simulink model "Stability2"  (R2024b)
settings: Solver=VariableStepAuto  StartTime=0.0  StopTime=3  RelTol=1e-3
settings Model: Creator=ADMIN  LastModifiedBy=ADMIN

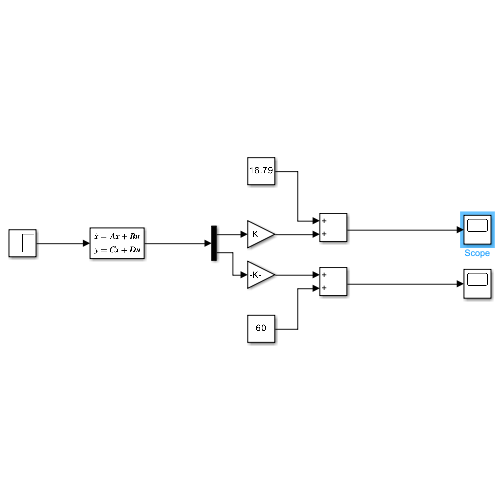
[thumbnail: Simulink's stored preview of the top-level diagram]
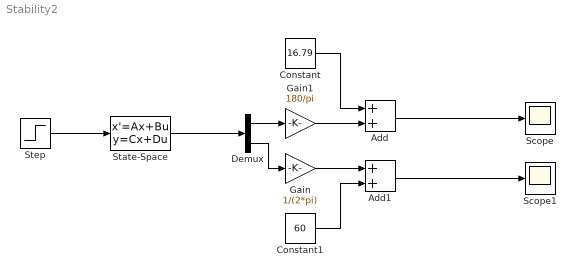
== system Stability2 ==
  Add : Sum
  Add1 : Sum
  Constant : Constant  Value=16.79
  Constant1 : Constant  Value=60
  Demux : Demux  Outputs=2
  Gain : Gain  Gain=1/(2*pi)
  Gain1 : Gain  Gain=180/pi
  Scope : Scope
  Scope1 : Scope
  State-Space : StateSpace  A=[0 1 ; -37.705 -2.617]  B=[0; 1]  C=[1 0; 0 1]  D=[0;0]  InitialCondition=0
  Step : Step  Time=0  Before=3.79  After=3.79  SampleTime=0
  wires:
  Step/1 -> State-Space/1
  Demux/1 -> Gain1/1
  State-Space/1 -> Demux/1
  Demux/2 -> Gain/1
  Gain/1 -> Add1/1
  Gain1/1 -> Add/2
  Constant/1 -> Add/1
  Constant1/1 -> Add1/2
  Add1/1 -> Scope1/1
  Add/1 -> Scope/1
